simulink model "gm_Encoder_Zynq"  (R2018a)
settings: Solver=ode3  StartTime=0.0  StopTime=SimulationsDauer  RelTol=1e-3  EnableMultiTasking=on
undefined symbols (not defined in the file or in its folder): DiscIntNeverNeededParam, IncPerTurn, n_max, OverSamplingFactor, OverSamplingFactorInverse, Periode, Phase_Delay_A, Phase_Delay_B, PolePair, T_mech, TestDrehzahl_rpm
libraries: dspswit3 x2, powerlib_meascontrol x2, hdlmdlgenlib x1, simulink_extras x1, powerlib x1
(part 1 of 2)
settings Model: Creator=Wendel_ELSYS  LastModifiedBy=Wendel
settings DataIOCC: LimitDataPoints=on  SaveFormat=Array
settings OptimizationCC: BlockReduction=off  ConditionallyExecuteInputs=off  DefaultParameterBehavior=Inlined  LifeSpan=inf
settings DebuggingCC: AlgebraicLoopMsg=error  InheritedTsInSrcMsg=none  ParameterOverflowMsg=none  SFUnexpectedBacktrackingDiag=warning  SFNoUnconditionalDefaultTransitionDiag=warning  SFExecutionAtInitializationDiag=none
settings HardwareCC: ProdBitPerPointer=32  ProdBitPerSizeT=32  ProdBitPerPtrDiffT=32  ProdLargestAtomicFloat=None  ProdIntDivRoundTo=Undefined  ProdEndianess=Unspecified  ProdWordSize=32  ProdHWDeviceType=ASIC/FPGA->ASIC/FPGA  ProdEqTarget=off
settings ModelReferenceCC: PropagateSignalLabelsOutOfModel=off
settings CodeAppCC: StateflowObjectComments=on
settings GRTTargetCC: TargetLangStandard=C89/C90 (ANSI)  GeneratePreprocessorConditionals=Disable all
settings ConfigComp: CovMetricSettings=dw  CovHtmlReporting=on  CovSaveCumulativeToWorkspaceVar=on  CovSaveSingleToWorkspaceVar=on  CovExternalEMLEnable=off
settings SimscapeCC: SimscapeNormalizeSystem=off

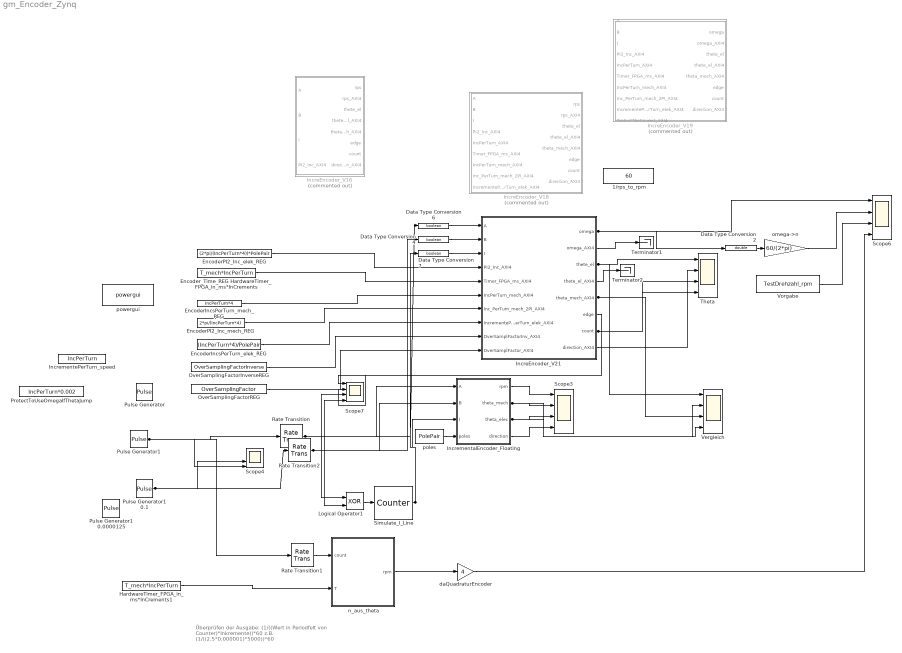
== system gm_Encoder_Zynq ==
  note: Überprüfen der Ausgabe:
      | (1/((Wert in Periodfelt von Counter)*Inkremente))*60
      | z.B. (1/((2.5*0.000001)*5000))*60
  1/rps_to_rpm : Constant  Value=60  OutDataTypeStr=double  SampleTime=T_mech
  Data Type Conversion2 : DataTypeConversion  OutDataTypeStr=double
  Data Type Conversion4 : DataTypeConversion  OutDataTypeStr=boolean
  Data Type Conversion6 : DataTypeConversion  OutDataTypeStr=boolean
  Data Type Conversion7 : DataTypeConversion  OutDataTypeStr=boolean
  "EncoderIncsPerTurn_elek_REG " : Constant  Value=(IncPerTurn*4)/PolePair  OutDataTypeStr=fixdt(0,16,0)  SampleTime=T_mech
  EncoderIncsPerTurn_mech_REG : Constant  Value=IncPerTurn*4  OutDataTypeStr=fixdt(0,16,0)  SampleTime=T_mech
  EncoderPI2_Inc_elek_REG : Constant  Value=(2*pi/(IncPerTurn*4))*PolePair  OutDataTypeStr=fixdt(0,24,24)  SampleTime=T_mech
  EncoderPI2_Inc_mech_REG : Constant  Value=2*pi/(IncPerTurn*4)  OutDataTypeStr=fixdt(0,24,24)  SampleTime=T_mech
  Encoder_Time_REG HardwareTimer_FPGA_in_ms*InCrements : Constant  Value=T_mech*IncPerTurn  OutDataTypeStr=fixdt(0,32,26)  SampleTime=T_mech
  HardwareTimer_FPGA_in_ms*InCrements1 : Constant  Value=T_mech*IncPerTurn  OutDataTypeStr=double  SampleTime=T_mech
  IncreEncoder_V16 : Subsystem  Commented=on  TreatAsAtomicUnit=on
  IncreEncoder_V18 : Subsystem  Commented=on  TreatAsAtomicUnit=on
  IncreEncoder_V19 : Subsystem  Commented=on  TreatAsAtomicUnit=on
  IncreEncoder_V21 : Subsystem  TreatAsAtomicUnit=on
  IncrementalEncoder_Floating : Subsystem
  IncrementePerTurn_speed : Constant  Value=IncPerTurn  OutDataTypeStr=fixdt(0,16,0)  SampleTime=T_mech
  Logical Operator1 : Logic  Operator=XOR  AllPortsSameDT=off  OutDataTypeStr=boolean
  OverSamplingFactorInverseREG : Constant  Value=OverSamplingFactorInverse  OutDataTypeStr=fixdt(0,16,15)  SampleTime=T_mech
  OverSamplingFactorREG : Constant  Value=OverSamplingFactor  OutDataTypeStr=fixdt(0,16,0)  SampleTime=T_mech
  ProtectToUseOmegaIfThetaJump : Constant  Value=IncPerTurn*0.002  OutDataTypeStr=uint16  SampleTime=T_mech
  Pulse Generator : DiscretePulseGenerator  PulseType=Time based  Period=0.01  PulseWidth=50  PhaseDelay=0.00000125  SampleTime=T_mech  VectorParams1D=off
  Pulse Generator1 : DiscretePulseGenerator  PulseType=Time based  Period=Periode  PulseWidth=50  PhaseDelay=Phase_Delay_A  SampleTime=T_mech  VectorParams1D=off
  Pulse Generator1 0.0000125 : DiscretePulseGenerator  PulseType=Time based  Period=0.01  PulseWidth=50  PhaseDelay=-0.00000125  SampleTime=T_mech  VectorParams1D=off
  Pulse Generator1 0.1 : DiscretePulseGenerator  PulseType=Time based  Period=Periode  PulseWidth=50  PhaseDelay=Phase_Delay_B  SampleTime=T_mech  VectorParams1D=off
  Rate Transition : RateTransition  Deterministic=off  OutPortSampleTime=T_mech
  Rate Transition1 : RateTransition  Deterministic=off  OutPortSampleTime=T_mech
  Rate Transition2 : RateTransition  Deterministic=off  OutPortSampleTime=T_mech
  Scope{3..4,6..7} (4 alike) : Scope  NumInputPorts=4
  Simulate_I_Line : dspswit3/Counter  Direction=Up  CountEvent=Either edge  CounterSize=User defined  MaxCount=IncPerTurn*4  InitialCount=0  Output=Hit  HitValue=IncPerTurn*4  ResetInput=off  SamplesPerFrame=1  Ts=1  CntDtype=double  HitDtype=Boolean
  Terminator1 : Terminator
  Terminator2 : Terminator
  Theta : Scope  NumInputPorts=4
  Vergleich : Scope  NumInputPorts=4
  Vorgabe : Constant  Value=TestDrehzahl_rpm
  "daQuadraturEncoder " : Gain  Gain=4
  n_aus_theta : Subsystem  TreatAsAtomicUnit=on
  omega->n : Gain  Gain=60/(2*pi)  OutDataTypeStr=double
  poles : Constant  Value=PolePair  OutDataTypeStr=uint8  SampleTime=-1
  powergui : powerlib/powergui  Priority=1  SimulationMode=Discrete  SampleTime=T_mech  frequency=60  Iterations=50  frequencyindice=0  Pbase=100e6  ErrMax=1e-4  UnitsV=kV  UnitsW=MW  buscounter=0  FunctionMessages=off  echomessages=off  EnableUseOfTLC=off  CurrentSourceSwitches=off  DisableSnubberDevices=off  DisableRonSwitches=off  DisableVfSwitches=off  DisplayEquations=off  SolverType=Tustin  Interpol=off  ExternalGateDelay=off  methode=off  Ts=0  x0status=blocks  SPID=off  SwTol=0  HookPort=off  RestoreLinks=warning  ResistiveCurrentMeasurement=off  Frange=[0:2:500]  Ylog=off  Xlog=on  ShowGrid=off  save=off  variable=ZData  structure=0  ZoomFFT=on  StartTime=0.0  cycles=1  DisplayStyle=1  fundamental=60  FreqAxis=off  MaxFrequency=1000  frequencyindicesteady=1  RmsSteady=1  display=off
  wires:
  OverSamplingFactorREG/1 -> IncreEncoder_V21/10(OverSamplFactor_AXI4)
  OverSamplingFactorInverseREG/1 -> IncreEncoder_V21/9(OverSamplFactorInv_AXI4)
  Vorgabe/1 -> Scope6/3
  "daQuadraturEncoder "/1 -> Scope6/4
  Pulse Generator1/1 -> Scope4/4, Rate Transition/1, Rate Transition1/1
  n_aus_theta/1(rpm) -> "daQuadraturEncoder "/1
  Rate Transition1/1 -> n_aus_theta/1(count)
  HardwareTimer_FPGA_in_ms*InCrements1/1 -> n_aus_theta/2(T)
  Data Type Conversion2/1 -> omega->n/1
  omega->n/1 -> Scope6/2
  "EncoderIncsPerTurn_elek_REG "/1 -> IncreEncoder_V21/8(IncrementePerTurn_elek_AXI4)
  EncoderPI2_Inc_mech_REG/1 -> IncreEncoder_V21/7(Inc_PerTurn_mech_2PI_AXI4)
  EncoderIncsPerTurn_mech_REG/1 -> IncreEncoder_V21/6(IncPerTurn_mech_AXI4)
  Encoder_Time_REG HardwareTimer_FPGA_in_ms*InCrements/1 -> IncreEncoder_V21/5(Timer_FPGA_ms_AXI4)
  IncreEncoder_V21/2(omega_AXI4) -> Terminator1/1
  IncreEncoder_V21/4(thete_el_AXI4) -> Terminator2/1
  IncreEncoder_V21/5(theta_mech_AXI4) -> Theta/3, Vergleich/3
  IncreEncoder_V21/3(thete_el) -> Vergleich/1, Theta/1
  EncoderPI2_Inc_elek_REG/1 -> IncreEncoder_V21/4(PI2_Inc_AXI4)
  poles/1 -> IncrementalEncoder_Floating/4(poles)
  IncrementalEncoder_Floating/4(direction) -> Scope3/4
  IncrementalEncoder_Floating/3(theta_elec) -> Scope3/3, Vergleich/2
  IncrementalEncoder_Floating/2(theta_mech) -> Scope3/2, Vergleich/4
  IncrementalEncoder_Floating/1(rpm) -> Scope3/1
  IncreEncoder_V21/7(count) -> Scope7/2, Theta/4
  IncreEncoder_V21/6(edge) -> Scope7/1
  IncreEncoder_V21/8(direction_AXI4) -> Theta/2
  IncreEncoder_V21/1(omega) -> Data Type Conversion2/1, Scope6/1
  Data Type Conversion7/1 -> IncreEncoder_V21/3(I)
  Data Type Conversion4/1 -> IncreEncoder_V21/2(B)
  Data Type Conversion6/1 -> IncreEncoder_V21/1(A)
  Rate Transition/1 -> Logical Operator1/1, IncrementalEncoder_Floating/1(A), Data Type Conversion6/1, Scope7/3
  Logical Operator1/1 -> Simulate_I_Line/1
  Simulate_I_Line/1 -> Data Type Conversion7/1, IncrementalEncoder_Floating/3(I)
  Rate Transition2/1 -> Data Type Conversion4/1, IncrementalEncoder_Floating/2(B), Scope7/4, Logical Operator1/2
  Pulse Generator1 0.1/1 -> Rate Transition2/1, Scope4/3

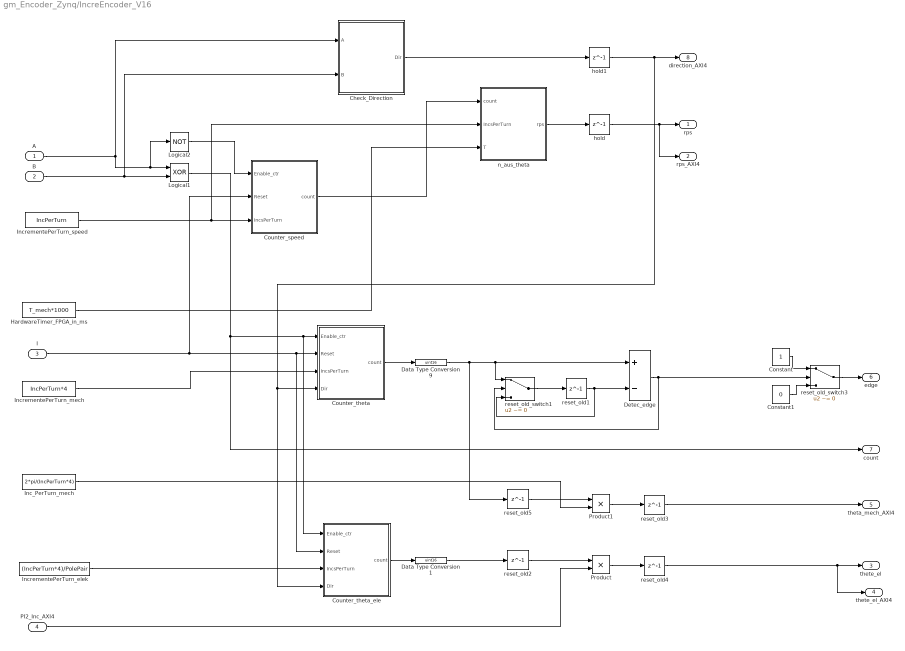
== system gm_Encoder_Zynq/IncreEncoder_V16 ==
  A : Inport
  B : Inport  Port=2
  I : Inport  Port=3
  PI2_Inc_AXI4 : Inport  Port=4
  Check_Direction : Subsystem  TreatAsAtomicUnit=on
  Constant : Constant  OutDataTypeStr=boolean  SampleTime=-1
  Constant1 : Constant  Value=0  OutDataTypeStr=boolean  SampleTime=-1
  Counter_speed : Subsystem  TreatAsAtomicUnit=on
  Counter_theta : Subsystem  TreatAsAtomicUnit=on
  Counter_theta_ele : Subsystem  TreatAsAtomicUnit=on
  Data Type Conversion1 : DataTypeConversion  OutDataTypeStr=uint16
  Data Type Conversion9 : DataTypeConversion  OutDataTypeStr=uint16
  Detec_edge : Sum  Inputs=+-  AccumDataTypeStr=uint8  OutDataTypeStr=uint8
  HardwareTimer_FPGA_in_ms : Constant  Value=T_mech*1000  OutDataTypeStr=fixdt(0,30,24)  SampleTime=T_mech
  Inc_PerTurn_mech : Constant  Value=2*pi/(IncPerTurn*4)  OutDataTypeStr=fixdt(0,24,24)  SampleTime=T_mech
  IncrementePerTurn_elek : Constant  Value=(IncPerTurn*4)/PolePair  OutDataTypeStr=fixdt(0,16,0)  SampleTime=T_mech
  IncrementePerTurn_mech : Constant  Value=IncPerTurn*4  OutDataTypeStr=fixdt(0,16,0)  SampleTime=T_mech
  IncrementePerTurn_speed : Constant  Value=IncPerTurn  OutDataTypeStr=fixdt(0,16,0)  SampleTime=T_mech
  Logical1 : Logic  Operator=XOR  AllPortsSameDT=off  OutDataTypeStr=boolean
  Logical2 : Logic  Operator=NOT  AllPortsSameDT=off  OutDataTypeStr=boolean
  Product : Product  OutDataTypeStr=fixdt(0,24,20)
  Product1 : Product  OutDataTypeStr=fixdt(0,24,20)
  hold : Delay  DelayLength=1
  hold1 : Delay  DelayLength=1
  n_aus_theta : Subsystem  TreatAsAtomicUnit=on
  reset_old{1..5} (5 alike) : Delay  DelayLength=1
  reset_old_switch1 : Switch  Criteria=u2 ~= 0
  reset_old_switch3 : Switch  Criteria=u2 ~= 0
  rps : Outport
  rps_AXI4 : Outport  Port=2
  thete_el : Outport  Port=3
  thete_el_AXI4 : Outport  Port=4
  theta_mech_AXI4 : Outport  Port=5
  edge : Outport  Port=6
  count : Outport  Port=7
  direction_AXI4 : Outport  Port=8
  wires:
  HardwareTimer_FPGA_in_ms/1 -> n_aus_theta/3(T)
  Logical2/1 -> Counter_speed/1(Enable_ctr)
  reset_old5/1 -> Product1/1
  reset_old2/1 -> Product/1
  Data Type Conversion1/1 -> reset_old2/1
  reset_old4/1 -> thete_el/1, thete_el_AXI4/1
  Counter_theta_ele/1(count) -> Data Type Conversion1/1
  PI2_Inc_AXI4/1 -> Product/2
  IncrementePerTurn_elek/1 -> Counter_theta_ele/3(IncsPerTurn)
  Data Type Conversion9/1 -> reset_old_switch1/1, Detec_edge/1, reset_old5/1
  n_aus_theta/1(rps) -> hold/1
  IncrementePerTurn_mech/1 -> Counter_theta/3(IncsPerTurn)
  Counter_speed/1(count) -> n_aus_theta/1(count)
  Logical1/1 -> Counter_theta/1(Enable_ctr), Counter_theta_ele/1(Enable_ctr), count/1
  Detec_edge/1 -> reset_old_switch1/2, reset_old_switch3/2
  Constant1/1 -> reset_old_switch3/3
  reset_old_switch3/1 -> edge/1
  Constant/1 -> reset_old_switch3/1
  Product/1 -> reset_old4/1
  Inc_PerTurn_mech/1 -> Product1/2
  Product1/1 -> reset_old3/1
  reset_old3/1 -> theta_mech_AXI4/1
  reset_old1/1 -> Detec_edge/2, reset_old_switch1/3
  reset_old_switch1/1 -> reset_old1/1
  Counter_theta/1(count) -> Data Type Conversion9/1
  hold1/1 -> direction_AXI4/1, Counter_theta/4(Dir), Counter_theta_ele/4(Dir)
  hold/1 -> rps/1, rps_AXI4/1
  Check_Direction/1(Dir) -> hold1/1
  IncrementePerTurn_speed/1 -> n_aus_theta/2(IncsPerTurn), Counter_speed/3(IncsPerTurn)
  I/1 -> Counter_theta/2(Reset), Counter_theta_ele/2(Reset), Counter_speed/2(Reset)
  B/1 -> Logical1/2, Check_Direction/2(B)
  A/1 -> Logical1/1, Logical2/1, Check_Direction/1(A)

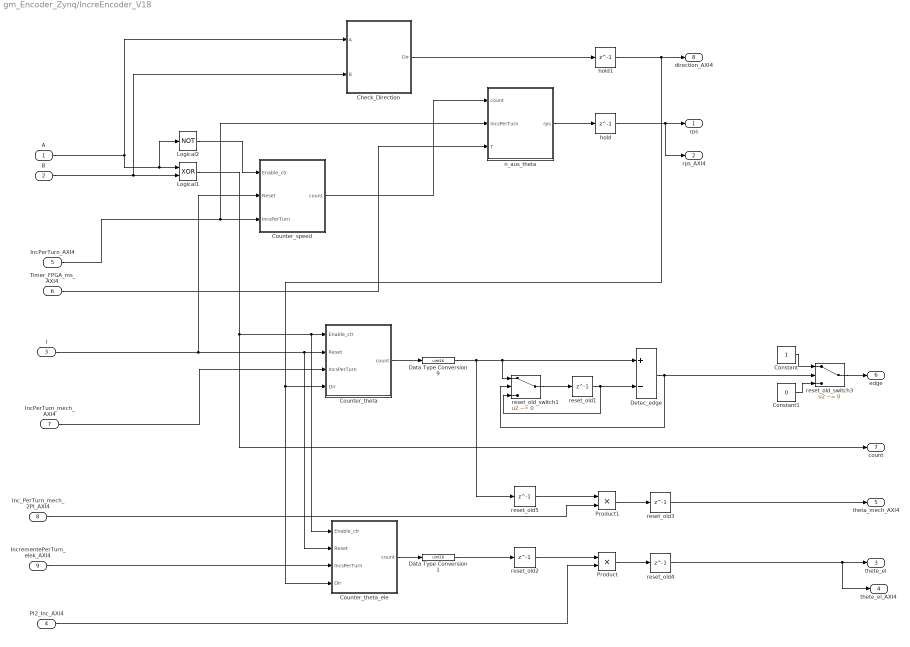
== system gm_Encoder_Zynq/IncreEncoder_V18 ==
  A : Inport
  B : Inport  Port=2
  I : Inport  Port=3
  PI2_Inc_AXI4 : Inport  Port=4
  IncPerTurn_AXI4 : Inport  Port=5
  Timer_FPGA_ms_AXI4 : Inport  Port=6
  IncPerTurn_mech_AXI4 : Inport  Port=7
  Inc_PerTurn_mech_2PI_AXI4 : Inport  Port=8
  IncrementePerTurn_elek_AXI4 : Inport  Port=9
  Check_Direction : Subsystem  TreatAsAtomicUnit=on
  Constant : Constant  OutDataTypeStr=boolean  SampleTime=-1
  Constant1 : Constant  Value=0  OutDataTypeStr=boolean  SampleTime=-1
  Counter_speed : Subsystem  TreatAsAtomicUnit=on
  Counter_theta : Subsystem  TreatAsAtomicUnit=on
  Counter_theta_ele : Subsystem  TreatAsAtomicUnit=on
  Data Type Conversion1 : DataTypeConversion  OutDataTypeStr=uint16
  Data Type Conversion9 : DataTypeConversion  OutDataTypeStr=uint16
  Detec_edge : Sum  Inputs=+-  AccumDataTypeStr=uint8  OutDataTypeStr=uint8
  Logical1 : Logic  Operator=XOR  AllPortsSameDT=off  OutDataTypeStr=boolean
  Logical2 : Logic  Operator=NOT  AllPortsSameDT=off  OutDataTypeStr=boolean
  Product : Product  OutDataTypeStr=fixdt(1,24,20)
  Product1 : Product  OutDataTypeStr=fixdt(1,24,20)
  hold : Delay  DelayLength=1
  hold1 : Delay  DelayLength=1
  n_aus_theta : Subsystem  TreatAsAtomicUnit=on
  reset_old{1..5} (5 alike) : Delay  DelayLength=1
  reset_old_switch1 : Switch  Criteria=u2 ~= 0
  reset_old_switch3 : Switch  Criteria=u2 ~= 0
  rps : Outport
  rps_AXI4 : Outport  Port=2
  thete_el : Outport  Port=3
  thete_el_AXI4 : Outport  Port=4
  theta_mech_AXI4 : Outport  Port=5
  edge : Outport  Port=6
  count : Outport  Port=7
  direction_AXI4 : Outport  Port=8
  wires:
  Timer_FPGA_ms_AXI4/1 -> n_aus_theta/3(T)
  Logical2/1 -> Counter_speed/1(Enable_ctr)
  reset_old5/1 -> Product1/1
  reset_old2/1 -> Product/1
  Data Type Conversion1/1 -> reset_old2/1
  reset_old4/1 -> thete_el/1, thete_el_AXI4/1
  Counter_theta_ele/1(count) -> Data Type Conversion1/1
  PI2_Inc_AXI4/1 -> Product/2
  IncrementePerTurn_elek_AXI4/1 -> Counter_theta_ele/3(IncsPerTurn)
  Data Type Conversion9/1 -> reset_old_switch1/1, Detec_edge/1, reset_old5/1
  n_aus_theta/1(rps) -> hold/1
  IncPerTurn_mech_AXI4/1 -> Counter_theta/3(IncsPerTurn)
  Counter_speed/1(count) -> n_aus_theta/1(count)
  Logical1/1 -> Counter_theta/1(Enable_ctr), Counter_theta_ele/1(Enable_ctr), count/1
  Detec_edge/1 -> reset_old_switch1/2, reset_old_switch3/2
  Constant1/1 -> reset_old_switch3/3
  reset_old_switch3/1 -> edge/1
  Constant/1 -> reset_old_switch3/1
  Product/1 -> reset_old4/1
  Inc_PerTurn_mech_2PI_AXI4/1 -> Product1/2
  Product1/1 -> reset_old3/1
  reset_old3/1 -> theta_mech_AXI4/1
  reset_old1/1 -> Detec_edge/2, reset_old_switch1/3
  reset_old_switch1/1 -> reset_old1/1
  Counter_theta/1(count) -> Data Type Conversion9/1
  hold1/1 -> direction_AXI4/1, Counter_theta/4(Dir), Counter_theta_ele/4(Dir)
  hold/1 -> rps/1, rps_AXI4/1
  Check_Direction/1(Dir) -> hold1/1
  IncPerTurn_AXI4/1 -> n_aus_theta/2(IncsPerTurn), Counter_speed/3(IncsPerTurn)
  I/1 -> Counter_theta/2(Reset), Counter_theta_ele/2(Reset), Counter_speed/2(Reset)
  B/1 -> Logical1/2, Check_Direction/2(B)
  A/1 -> Logical1/1, Logical2/1, Check_Direction/1(A)

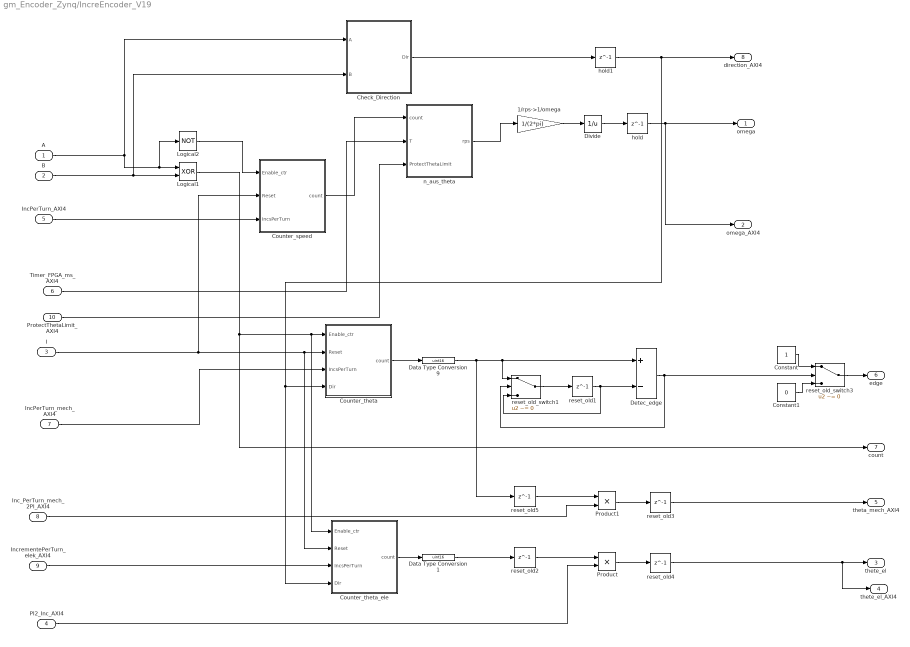
== system gm_Encoder_Zynq/IncreEncoder_V19 ==
  A : Inport
  B : Inport  Port=2
  I : Inport  Port=3
  PI2_Inc_AXI4 : Inport  Port=4
  IncPerTurn_AXI4 : Inport  Port=5
  Timer_FPGA_ms_AXI4 : Inport  Port=6
  IncPerTurn_mech_AXI4 : Inport  Port=7
  Inc_PerTurn_mech_2PI_AXI4 : Inport  Port=8
  IncrementePerTurn_elek_AXI4 : Inport  Port=9
  ProtectThetaLimit_AXI4 : Inport  Port=10
  1/rps->1/omega : Gain  Gain=1/(2*pi)  OutDataTypeStr=fixdt(1,24,18)
  Check_Direction : Subsystem  TreatAsAtomicUnit=on
  Constant : Constant  OutDataTypeStr=boolean  SampleTime=-1
  Constant1 : Constant  Value=0  OutDataTypeStr=boolean  SampleTime=-1
  Counter_speed : Subsystem  TreatAsAtomicUnit=on
  Counter_theta : Subsystem  TreatAsAtomicUnit=on
  Counter_theta_ele : Subsystem  TreatAsAtomicUnit=on
  Data Type Conversion1 : DataTypeConversion  OutDataTypeStr=uint16
  Data Type Conversion9 : DataTypeConversion  OutDataTypeStr=uint16
  Detec_edge : Sum  Inputs=+-  AccumDataTypeStr=uint8  OutDataTypeStr=uint8
  Divide : Math  Operator=reciprocal  OutDataTypeStr=fixdt(1,24,11)  RndMeth=Zero  SaturateOnIntegerOverflow=on
  Logical1 : Logic  Operator=XOR  AllPortsSameDT=off  OutDataTypeStr=boolean
  Logical2 : Logic  Operator=NOT  AllPortsSameDT=off  OutDataTypeStr=boolean
  Product : Product  OutDataTypeStr=fixdt(1,24,20)
  Product1 : Product  OutDataTypeStr=fixdt(1,24,20)
  hold : Delay  DelayLength=1
  hold1 : Delay  DelayLength=1
  n_aus_theta : Subsystem  TreatAsAtomicUnit=on
  reset_old{1..5} (5 alike) : Delay  DelayLength=1
  reset_old_switch1 : Switch  Criteria=u2 ~= 0
  reset_old_switch3 : Switch  Criteria=u2 ~= 0
  omega : Outport
  omega_AXI4 : Outport  Port=2
  thete_el : Outport  Port=3
  thete_el_AXI4 : Outport  Port=4
  theta_mech_AXI4 : Outport  Port=5
  edge : Outport  Port=6
  count : Outport  Port=7
  direction_AXI4 : Outport  Port=8
  wires:
  ProtectThetaLimit_AXI4/1 -> n_aus_theta/3(ProtectThetaLimit)
  1/rps->1/omega/1 -> Divide/1
  Divide/1 -> hold/1
  Timer_FPGA_ms_AXI4/1 -> n_aus_theta/2(T)
  Logical2/1 -> Counter_speed/1(Enable_ctr)
  reset_old5/1 -> Product1/1
  reset_old2/1 -> Product/1
  Data Type Conversion1/1 -> reset_old2/1
  reset_old4/1 -> thete_el/1, thete_el_AXI4/1
  Counter_theta_ele/1(count) -> Data Type Conversion1/1
  PI2_Inc_AXI4/1 -> Product/2
  IncrementePerTurn_elek_AXI4/1 -> Counter_theta_ele/3(IncsPerTurn)
  Data Type Conversion9/1 -> reset_old_switch1/1, Detec_edge/1, reset_old5/1
  n_aus_theta/1(rps) -> 1/rps->1/omega/1
  IncPerTurn_mech_AXI4/1 -> Counter_theta/3(IncsPerTurn)
  Counter_speed/1(count) -> n_aus_theta/1(count)
  Logical1/1 -> Counter_theta/1(Enable_ctr), Counter_theta_ele/1(Enable_ctr), count/1
  Detec_edge/1 -> reset_old_switch1/2, reset_old_switch3/2
  Constant1/1 -> reset_old_switch3/3
  reset_old_switch3/1 -> edge/1
  Constant/1 -> reset_old_switch3/1
  Product/1 -> reset_old4/1
  Inc_PerTurn_mech_2PI_AXI4/1 -> Product1/2
  Product1/1 -> reset_old3/1
  reset_old3/1 -> theta_mech_AXI4/1
  reset_old1/1 -> Detec_edge/2, reset_old_switch1/3
  reset_old_switch1/1 -> reset_old1/1
  Counter_theta/1(count) -> Data Type Conversion9/1
  hold1/1 -> direction_AXI4/1, Counter_theta/4(Dir), Counter_theta_ele/4(Dir)
  hold/1 -> omega/1, omega_AXI4/1
  Check_Direction/1(Dir) -> hold1/1
  IncPerTurn_AXI4/1 -> Counter_speed/3(IncsPerTurn)
  I/1 -> Counter_theta/2(Reset), Counter_theta_ele/2(Reset), Counter_speed/2(Reset)
  B/1 -> Logical1/2, Check_Direction/2(B)
  A/1 -> Logical1/1, Logical2/1, Check_Direction/1(A)

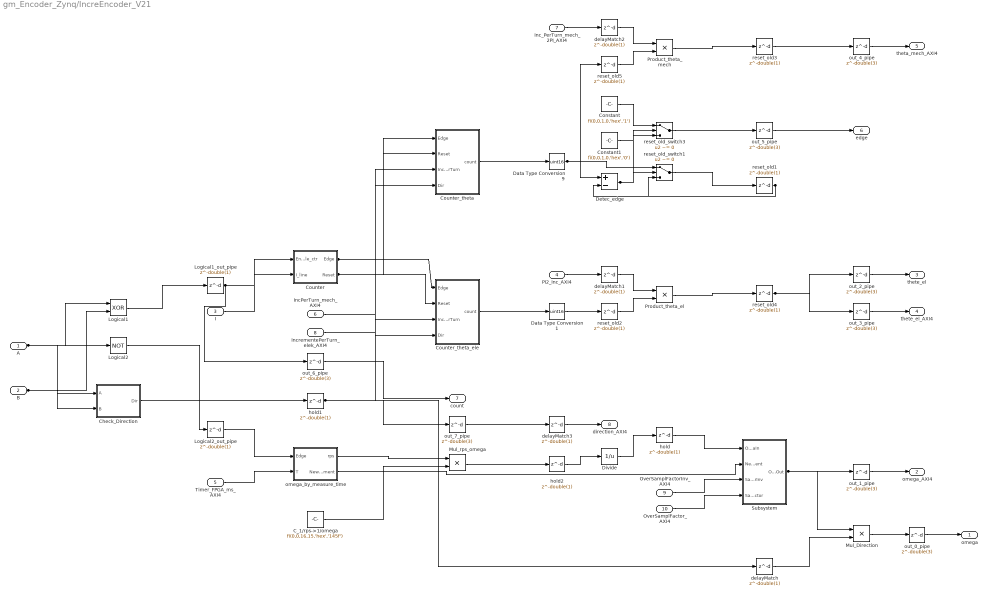
== system gm_Encoder_Zynq/IncreEncoder_V21 ==
  A : Inport  OutDataTypeStr=boolean  PortDimensions=1  SampleTime=2e-08
  B : Inport  Port=2  OutDataTypeStr=boolean  PortDimensions=1  SampleTime=2e-08
  I : Inport  Port=3  OutDataTypeStr=boolean  PortDimensions=1  SampleTime=2e-08
  PI2_Inc_AXI4 : Inport  Port=4  OutDataTypeStr=fixdt(0, 24, 24)  PortDimensions=1  SampleTime=2e-08
  Timer_FPGA_ms_AXI4 : Inport  Port=5  OutDataTypeStr=fixdt(0, 32, 26)  PortDimensions=1  SampleTime=2e-08
  IncPerTurn_mech_AXI4 : Inport  Port=6  OutDataTypeStr=uint16  PortDimensions=1  SampleTime=2e-08
  Inc_PerTurn_mech_2PI_AXI4 : Inport  Port=7  OutDataTypeStr=fixdt(0, 24, 24)  PortDimensions=1  SampleTime=2e-08
  IncrementePerTurn_elek_AXI4 : Inport  Port=8  OutDataTypeStr=uint16  PortDimensions=1  SampleTime=2e-08
  OverSamplFactorInv_AXI4 : Inport  Port=9  OutDataTypeStr=fixdt(0, 16, 15)  PortDimensions=1  SampleTime=2e-08
  OverSamplFactor_AXI4 : Inport  Port=10  OutDataTypeStr=uint16  PortDimensions=1  SampleTime=2e-08
  C_1/rps->1/omega : Constant  Value=fi(0,0,16,15,'hex','145f')  OutDataTypeStr=fixdt(0, 16, 15)  SampleTime=-1
  Check_Direction : Subsystem
  Constant : Constant  Value=fi(0,0,1,0,'hex','1')  OutDataTypeStr=boolean  SampleTime=-1
  Constant1 : Constant  Value=fi(0,0,1,0,'hex','0')  OutDataTypeStr=boolean  SampleTime=-1
  Counter : Subsystem
  Counter_theta : Subsystem
  Counter_theta_ele : Subsystem
  Data Type Conversion1 : DataTypeConversion  OutDataTypeStr=uint16  SampleTime=2e-08
  Data Type Conversion9 : DataTypeConversion  OutDataTypeStr=uint16  SampleTime=2e-08
  Detec_edge : Sum  Inputs=+-  AccumDataTypeStr=uint8  OutDataTypeStr=uint8  SampleTime=2e-08
  Divide : Math  Operator=reciprocal  OutDataTypeStr=fixdt(1,24,11)  RndMeth=Zero  SaturateOnIntegerOverflow=on
  Logical1 : Logic  Operator=XOR  AllPortsSameDT=off  OutDataTypeStr=boolean  SampleTime=2e-08
  Logical1_out_pipe : Delay  DelayLength=double(1)  InitialCondition=0  InputProcessing=Inherited  SampleTime=2e-08
  Logical2 : Logic  Operator=NOT  Inputs=1  AllPortsSameDT=off  OutDataTypeStr=boolean  SampleTime=2e-08
  Logical2_out_pipe : Delay  DelayLength=double(1)  InitialCondition=0  InputProcessing=Inherited  SampleTime=2e-08
  Mul_Direction : Product  Inputs=**  OutDataTypeStr=fixdt(1, 24, 11)  SampleTime=2e-08  SaturateOnIntegerOverflow=on  RndMeth=Zero
  Mul_rps_omega : Product  Inputs=**  OutDataTypeStr=fixdt(0, 32, 26)  SampleTime=2e-08  SaturateOnIntegerOverflow=on  RndMeth=Zero
  Product_theta_el : Product  Inputs=**  OutDataTypeStr=fixdt(1, 24, 20)  SampleTime=2e-08
  Product_theta_mech : Product  Inputs=**  OutDataTypeStr=fixdt(1, 24, 20)  SampleTime=2e-08
  Subsystem : Subsystem
  delayMatch{,1..3} (4 alike) : Delay  DelayLength=double(1)  InitialCondition=0  InputProcessing=Inherited  SampleTime=2e-08
  hold : Delay  DelayLength=double(1)  InitialCondition=0  InputProcessing=Inherited  SampleTime=2e-08
  hold1 : Delay  DelayLength=double(1)  InitialCondition=0  InputProcessing=Inherited  SampleTime=2e-08
  hold2 : Delay  DelayLength=double(1)  InitialCondition=0  InputProcessing=Inherited  SampleTime=2e-08
  omega_by_measure_time : Subsystem
  out_0_pipe : Delay  DelayLength=double(3)  InitialCondition=0  InputProcessing=Inherited  SampleTime=2e-08
  out_1_pipe : Delay  DelayLength=double(3)  InitialCondition=0  InputProcessing=Inherited  SampleTime=2e-08
  out_2_pipe : Delay  DelayLength=double(3)  InitialCondition=0  InputProcessing=Inherited  SampleTime=2e-08
  out_3_pipe : Delay  DelayLength=double(3)  InitialCondition=0  InputProcessing=Inherited  SampleTime=2e-08
  out_4_pipe : Delay  DelayLength=double(3)  InitialCondition=0  InputProcessing=Inherited  SampleTime=2e-08
  out_5_pipe : Delay  DelayLength=double(3)  InitialCondition=0  InputProcessing=Inherited  SampleTime=2e-08
  out_6_pipe : Delay  DelayLength=double(3)  InitialCondition=0  InputProcessing=Inherited  SampleTime=2e-08
  out_7_pipe : Delay  DelayLength=double(3)  InitialCondition=0  InputProcessing=Inherited  SampleTime=2e-08
  reset_old{1..5} (5 alike) : Delay  DelayLength=double(1)  InitialCondition=0  InputProcessing=Inherited  SampleTime=2e-08
  reset_old_switch1 : Switch  Criteria=u2 ~= 0  Threshold=double(0)  OutDataTypeStr=uint16  SampleTime=2e-08
  reset_old_switch3 : Switch  Criteria=u2 ~= 0  Threshold=double(0)  OutDataTypeStr=boolean  SampleTime=2e-08
  omega : Outport
  omega_AXI4 : Outport  Port=2
  thete_el : Outport  Port=3
  thete_el_AXI4 : Outport  Port=4
  theta_mech_AXI4 : Outport  Port=5
  edge : Outport  Port=6
  count : Outport  Port=7
  direction_AXI4 : Outport  Port=8
  wires:
  A/1 -> Logical2/1, Logical1/1, Check_Direction/1(A)
  B/1 -> Logical1/2, Check_Direction/2(B)
  I/1 -> Counter/2(I_line)
  delayMatch1/1 -> Product_theta_el/1
  Timer_FPGA_ms_AXI4/1 -> omega_by_measure_time/2(T)
  IncPerTurn_mech_AXI4/1 -> Counter_theta/3(IncsPerTurn)
  delayMatch2/1 -> Product_theta_mech/1
  IncrementePerTurn_elek_AXI4/1 -> Counter_theta_ele/3(IncsPerTurn)
  OverSamplFactorInv_AXI4/1 -> Subsystem/3(SamplingFactorInv)
  OverSamplFactor_AXI4/1 -> Subsystem/4(SamplingFactor)
  C_1/rps->1/omega/1 -> Mul_rps_omega/2
  Check_Direction/1(Dir) -> hold1/1
  Constant/1 -> reset_old_switch3/1
  Constant1/1 -> reset_old_switch3/3
  Counter/1(Edge) -> Counter_theta_ele/1(Edge), Counter_theta/1(Edge)
  Counter/2(Reset) -> Counter_theta_ele/2(Reset), Counter_theta/2(Reset)
  Counter_theta/1(count) -> Data Type Conversion9/1
  Counter_theta_ele/1(count) -> Data Type Conversion1/1
  Data Type Conversion1/1 -> reset_old2/1
  Data Type Conversion9/1 -> reset_old5/1, reset_old_switch1/1, Detec_edge/1
  Divide/1 -> hold/1
  Logical1_out_pipe/1 -> out_6_pipe/1, Counter/1(Enable_ctr)
  Logical2_out_pipe/1 -> omega_by_measure_time/1(Edge)
  Mul_Direction/1 -> out_0_pipe/1
  Mul_rps_omega/1 -> hold2/1
  Product_theta_el/1 -> reset_old4/1
  Product_theta_mech/1 -> reset_old3/1
  Subsystem/1(OmegaOut) -> Mul_Direction/1, out_1_pipe/1
  hold/1 -> Subsystem/1("OmegaIn ")
  delayMatch/1 -> Mul_Direction/2
  hold2/1 -> Divide/1
  omega_by_measure_time/1(rps) -> Mul_rps_omega/1
  omega_by_measure_time/2(NewMeasurement) -> Subsystem/2(NewMeasurement)
  reset_old2/1 -> Product_theta_el/2
  reset_old3/1 -> out_4_pipe/1
  reset_old4/1 -> out_3_pipe/1, out_2_pipe/1
  reset_old5/1 -> Product_theta_mech/2
  reset_old_switch3/1 -> out_5_pipe/1
  out_0_pipe/1 -> omega/1
  out_1_pipe/1 -> omega_AXI4/1
  out_2_pipe/1 -> thete_el/1
  out_3_pipe/1 -> thete_el_AXI4/1
  out_4_pipe/1 -> theta_mech_AXI4/1
  out_5_pipe/1 -> edge/1
  out_6_pipe/1 -> count/1
  delayMatch3/1 -> direction_AXI4/1
  Logical1/1 -> Logical1_out_pipe/1
  Logical2/1 -> Logical2_out_pipe/1
  hold1/1 -> delayMatch/1, out_7_pipe/1, Counter_theta_ele/4(Dir), Counter_theta/4(Dir)
  PI2_Inc_AXI4/1 -> delayMatch1/1
  Inc_PerTurn_mech_2PI_AXI4/1 -> delayMatch2/1
  out_7_pipe/1 -> delayMatch3/1
  reset_old_switch1/1 -> reset_old1/1
  reset_old1/1 -> reset_old_switch1/3, Detec_edge/2
  Detec_edge/1 -> reset_old_switch1/2, reset_old_switch3/2

== system gm_Encoder_Zynq/IncrementalEncoder_Floating ==
  A : Inport
  B : Inport  Port=2
  I : Inport  Port=3
  poles : Inport  Port=4
  Add : Sum  Inputs=+-  OutDataTypeStr=fixdt(1,16,0)
  Counter3 : dspswit3/Counter  Direction=Up  CountEvent=Either edge  CounterSize=User defined  MaxCount=IncPerTurn*4  InitialCount=0  Output=Count  HitValue=32  ResetInput=on  SamplesPerFrame=1  Ts=1  CntDtype=double  HitDtype=Logical
  CutTheta_0_2PI : Subsystem
  Edge Detector2 : powerlib_meascontrol/Logic/Edge Detector  model=Rising  ic=0  Ts=-1
      settings: SourceProductName=Simscape Power Systems  SourceProductBaseCode=PS
  Edge Detector3 : powerlib_meascontrol/Logic/Edge Detector  model=Rising  ic=0  Ts=-1
      settings: SourceProductName=Simscape Power Systems  SourceProductBaseCode=PS
  Logical Operator1 : Logic  Operator=XOR  AllPortsSameDT=off  OutDataTypeStr=boolean
  Logical Operator3 : Logic  AllPortsSameDT=off  OutDataTypeStr=boolean
  Logical Operator4 : Logic  Operator=NOT  AllPortsSameDT=off  OutDataTypeStr=boolean
  Logical Operator5 : Logic  AllPortsSameDT=off  OutDataTypeStr=boolean
  Logical Operator6 : Logic  Operator=NOT  AllPortsSameDT=off  OutDataTypeStr=boolean
  Product : Product
  S-R Flip-Flop1 : simulink_extras/Flip Flops/S-R Flip-Flop  initial_condition=0
  Scope1 : Scope  NumInputPorts=4
  cut_theta_2pi : Gain  Gain=(2*pi)/IncPerTurn
  cut_theta_2pi1 : Gain  Gain=(2*pi)/IncPerTurn
  n_aus_theta_v4 : Subsystem
  rpm : Outport
  theta_mech : Outport  Port=2
  theta_elec : Outport  Port=3
  direction : Outport  Port=4
  wires:
  Add/1 -> direction/1
  B/1 -> Logical Operator1/2, Logical Operator4/1, Edge Detector3/1
  A/1 -> Logical Operator1/1, Edge Detector2/1, Logical Operator6/1
  S-R Flip-Flop1/2 -> Add/2
  S-R Flip-Flop1/1 -> Add/1
  Logical Operator5/1 -> S-R Flip-Flop1/2
  Logical Operator6/1 -> Logical Operator5/2
  Edge Detector3/1 -> Logical Operator5/1
  Logical Operator3/1 -> S-R Flip-Flop1/1
  Logical Operator4/1 -> Logical Operator3/2
  Edge Detector2/1 -> Logical Operator3/1
  CutTheta_0_2PI/1(Out1) -> theta_elec/1
  cut_theta_2pi1/1 -> CutTheta_0_2PI/1(In1)
  poles/1 -> Product/2
  Product/1 -> cut_theta_2pi1/1
  cut_theta_2pi/1 -> theta_mech/1, n_aus_theta_v4/1(theta), Scope1/2
  Logical Operator1/1 -> Counter3/1, Scope1/4
  n_aus_theta_v4/1(n) -> rpm/1
  Counter3/1 -> Scope1/1, Product/1, cut_theta_2pi/1
  I/1 -> Counter3/2

== system gm_Encoder_Zynq/n_aus_theta ==
  count : Inport
  T : Inport  Port=2
  1/rps->1/omega : Gain  Gain=1/(2*pi)  OutDataTypeStr=double
  Add : Sum  Inputs=+-
  Add1 : Sum
  Constant : Constant  Value=0  OutDataTypeStr=double  SampleTime=-1
  Constant1 : Constant  Value=0  OutDataTypeStr=double  SampleTime=-1
  Constant2 : Constant  Value=0  OutDataTypeStr=double  SampleTime=-1
  Divide1 : Product  Inputs=/
  ProtectOverflow_T_count : Switch  Threshold=50
  ProtectOverflow_rps : Switch  Threshold=50  OutDataTypeStr=double
  Scope1 : Scope  NumInputPorts=4
  Scope2 : Scope  NumInputPorts=4
  T_count : Delay  DelayLength=1
  T_count_switch : Switch  Criteria=u2 ~= 0
  count_old : Delay  DelayLength=1
  count_old_switch : Switch  Criteria=u2 ~= 0
  speed_old : Delay  DelayLength=1
  speed_old_switch : Switch  Criteria=u2 ~= 0
  rpm : Outport
  wires:
  Divide1/1 -> rpm/1
  1/rps->1/omega/1 -> Divide1/1
  T_count_switch/1 -> ProtectOverflow_T_count/3, ProtectOverflow_T_count/2, Scope1/2, ProtectOverflow_rps/2
  count/1 -> count_old_switch/1, Add/1
  Add1/1 -> T_count_switch/3, speed_old_switch/1, Scope2/2
  T_count/1 -> Add1/2, Scope1/4
  ProtectOverflow_T_count/1 -> T_count/1
  T/1 -> Add1/1, Scope2/4
  speed_old/1 -> speed_old_switch/3
  speed_old_switch/1 -> speed_old/1, Scope2/3, ProtectOverflow_rps/3
  Constant2/1 -> ProtectOverflow_rps/1
  ProtectOverflow_rps/1 -> Scope2/1, 1/rps->1/omega/1
  Constant1/1 -> ProtectOverflow_T_count/1
  Add/1 -> T_count_switch/2, Scope1/1, count_old_switch/2, speed_old_switch/2
  Constant/1 -> T_count_switch/1
  count_old/1 -> Add/2, count_old_switch/3
  count_old_switch/1 -> count_old/1

== system gm_Encoder_Zynq/IncreEncoder_V16/Check_Direction ==
  A : Inport
  B : Inport  Port=2
  Add : Sum  Inputs=+-  AccumDataTypeStr=fixdt(1,4,0)  OutDataTypeStr=fixdt(1,4,0)
  Add1 : Sum  Inputs=+-  AccumDataTypeStr=fixdt(1,4,0)  OutDataTypeStr=fixdt(1,4,0)
  Add2 : Sum  AccumDataTypeStr=fixdt(1,4,0)  OutDataTypeStr=fixdt(1,4,0)
  Change : Sum  AccumDataTypeStr=fixdt(1,4,0)  OutDataTypeStr=fixdt(1,4,0)
  Change1 : Delay  DelayLength=1
  Save_Direction : Switch  Criteria=u2 ~= 0  Threshold=0.1  OutDataTypeStr=Inherit: Inherit via back propagation
  Scope6 : Scope  NumInputPorts=4
  T_count_switch : Switch  Threshold=1  OutDataTypeStr=Inherit: Inherit via back propagation
  TrnLeft : Sum  Inputs=+-  AccumDataTypeStr=fixdt(1,4,0)  OutDataTypeStr=fixdt(1,4,0)
  TrnRight : Sum  Inputs=+-  AccumDataTypeStr=fixdt(1,4,0)  OutDataTypeStr=fixdt(1,4,0)
  TurnLeft : Constant  Value=-1  OutDataTypeStr=fixdt(1,4,0)  SampleTime=-1
  TurnRight : Constant  OutDataTypeStr=fixdt(1,4,0)  SampleTime=-1
  count_old : Delay  DelayLength=1
  count_old1 : Delay  DelayLength=1
  count_old2 : Delay  DelayLength=1
  count_old_switch : Switch  Criteria=u2 ~= 0  OutDataTypeStr=Inherit: Inherit via back propagation
  count_old_switch1 : Switch  Criteria=u2 ~= 0  OutDataTypeStr=Inherit: Inherit via back propagation
  new_value : Delay  DelayLength=1
  nothing : Constant  Value=0  OutDataTypeStr=fixdt(1,4,0)  SampleTime=-1
  nothing1 : Constant  Value=0  OutDataTypeStr=fixdt(1,4,0)  SampleTime=-1
  speed_old_switch : Switch  Threshold=1  OutDataTypeStr=Inherit: Inherit via back propagation
  Dir : Outport
  wires:
  count_old2/1 -> Dir/1, Save_Direction/3
  Change1/1 -> Save_Direction/2, Scope6/3
  Change/1 -> Change1/1
  Add2/1 -> new_value/1, Scope6/4
  speed_old_switch/1 -> Add2/2, Change/2
  nothing1/1 -> T_count_switch/3
  nothing/1 -> speed_old_switch/3
  TurnLeft/1 -> speed_old_switch/1
  TrnLeft/1 -> Scope6/2, speed_old_switch/2
  new_value/1 -> Save_Direction/1
  TrnRight/1 -> T_count_switch/2, Scope6/1
  Add1/1 -> count_old_switch1/2, TrnLeft/1
  count_old1/1 -> Add1/2, count_old_switch1/3
  count_old_switch1/1 -> count_old1/1
  B/1 -> count_old_switch1/1, Add1/1, TrnRight/2
  Save_Direction/1 -> count_old2/1
  T_count_switch/1 -> Add2/1, Change/1
  Add/1 -> count_old_switch/2, TrnRight/1
  TurnRight/1 -> T_count_switch/1
  count_old/1 -> Add/2, count_old_switch/3
  count_old_switch/1 -> count_old/1
  A/1 -> count_old_switch/1, Add/1, TrnLeft/2

== system gm_Encoder_Zynq/IncreEncoder_V16/Counter_speed ==
  note: Count
  note: Reset
  note: Check if count is to big
  note: Check if count is to small
  note: 1 for one cycle if edge recognized
  Enable_ctr : Inport
  Reset : Inport  Port=2
  IncsPerTurn : Inport  Port=3
  Add1 : Sum  AccumDataTypeStr=int16  OutDataTypeStr=uint16
  Constant1 : Constant  Value=0  OutDataTypeStr=uint16  SampleTime=-1
  Constant2 : Constant  OutDataTypeStr=int8  SampleTime=-1
  Constant3 : Constant  Value=0  OutDataTypeStr=int8  SampleTime=-1
  Constant4 : Constant  Value=10  OutDataTypeStr=uint16  SampleTime=-1
  Detec_edge : Sum  Inputs=+-  AccumDataTypeStr=int8  OutDataTypeStr=int8
  Relational Operator : RelationalOperator  OutDataTypeStr=boolean  RndMeth=Nearest
  Reset_flag : Sum  Inputs=+-  AccumDataTypeStr=uint8  OutDataTypeStr=uint8
  Reset_when_overflow : Sum
  Resett_switch1 : Switch  Criteria=u2 ~= 0
  Resett_switch2 : Switch  Criteria=u2 ~= 0
  reset_old{,1..3} (4 alike) : Delay  DelayLength=1
  reset_old_switch : Switch  Criteria=u2 ~= 0
  reset_old_switch1 : Switch  Criteria=u2 ~= 0
  speed_old_switch1 : Switch  Threshold=1
  count : Outport
  wires:
  reset_old3/1 -> Relational Operator/2
  Resett_switch2/1 -> Resett_switch1/3
  IncsPerTurn/1 -> Reset_when_overflow/2
  Constant1/1 -> Resett_switch1/1, Resett_switch2/1
  Relational Operator/1 -> Resett_switch1/2
  Resett_switch1/1 -> reset_old2/1
  Reset_when_overflow/1 -> reset_old3/1
  Constant4/1 -> Reset_when_overflow/1
  Constant2/1 -> speed_old_switch1/1
  Constant3/1 -> speed_old_switch1/3
  speed_old_switch1/1 -> Add1/1
  reset_old2/1 -> count/1, Add1/2, Relational Operator/1
  Add1/1 -> Resett_switch2/3
  Detec_edge/1 -> reset_old_switch1/2, speed_old_switch1/2  "1 for one cycle if edge recognized"
  reset_old1/1 -> Detec_edge/2, reset_old_switch1/3
  reset_old_switch1/1 -> reset_old1/1
  Enable_ctr/1 -> reset_old_switch1/1, Detec_edge/1
  Reset_flag/1 -> Resett_switch2/2, reset_old_switch/2
  reset_old/1 -> Reset_flag/2, reset_old_switch/3
  reset_old_switch/1 -> reset_old/1
  Reset/1 -> reset_old_switch/1, Reset_flag/1

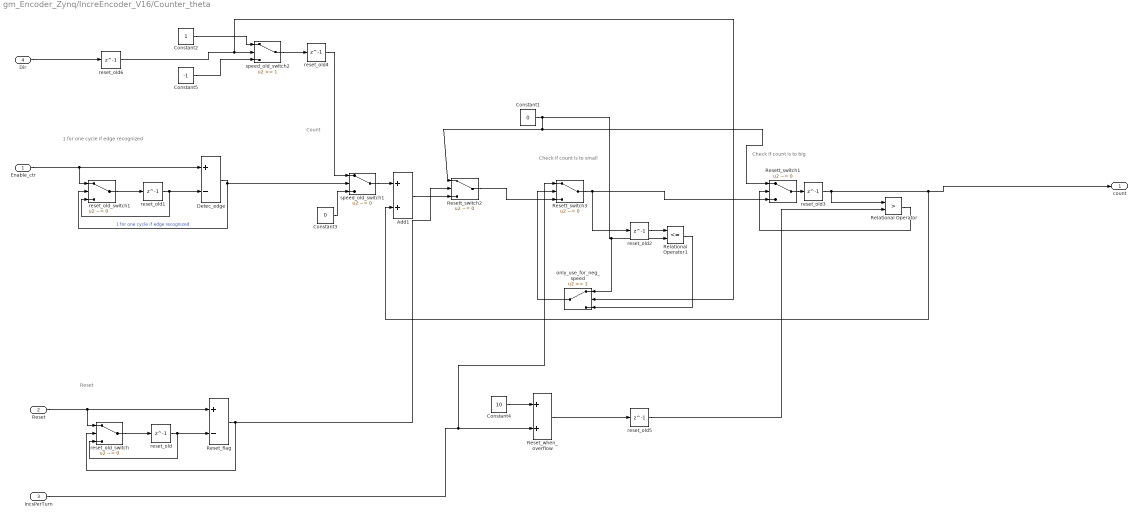
== system gm_Encoder_Zynq/IncreEncoder_V16/Counter_theta ==
  note: Check if count is to small
  note: Check if count is to big
  note: Count
  note: Reset
  note: 1 for one cycle if edge recognized
  Enable_ctr : Inport
  Reset : Inport  Port=2
  IncsPerTurn : Inport  Port=3
  Dir : Inport  Port=4
  Add1 : Sum  AccumDataTypeStr=int16  OutDataTypeStr=int16
  Constant1 : Constant  Value=0  OutDataTypeStr=int16  SampleTime=-1
  Constant2 : Constant  OutDataTypeStr=int16  SampleTime=-1
  Constant3 : Constant  Value=0  OutDataTypeStr=int16  SampleTime=-1
  Constant4 : Constant  Value=10  OutDataTypeStr=int16  SampleTime=-1
  Constant5 : Constant  Value=-1  OutDataTypeStr=int16  SampleTime=-1
  Detec_edge : Sum  Inputs=+-  AccumDataTypeStr=int8  OutDataTypeStr=int8
  Relational Operator : RelationalOperator  Operator=>  OutDataTypeStr=boolean  RndMeth=Nearest
  Relational Operator1 : RelationalOperator  Operator=<=  OutDataTypeStr=boolean  RndMeth=Nearest
  Reset_flag : Sum  Inputs=+-  AccumDataTypeStr=uint8  OutDataTypeStr=uint8
  Reset_when_overflow : Sum  OutDataTypeStr=int16
  Resett_switch1 : Switch  Criteria=u2 ~= 0  OutDataTypeStr=int16
  Resett_switch2 : Switch  Criteria=u2 ~= 0  OutDataTypeStr=int16
  Resett_switch3 : Switch  Criteria=u2 ~= 0  OutDataTypeStr=int16
  only_use_for_neg_speed : Switch  Threshold=1
  reset_old{,1..6} (7 alike) : Delay  DelayLength=1
  reset_old_switch : Switch  Criteria=u2 ~= 0
  reset_old_switch1 : Switch  Criteria=u2 ~= 0
  speed_old_switch1 : Switch  Criteria=u2 ~= 0
  speed_old_switch2 : Switch  Threshold=1
  count : Outport
  wires:
  reset_old6/1 -> speed_old_switch2/2, only_use_for_neg_speed/2
  reset_old5/1 -> Relational Operator/2
  reset_old4/1 -> speed_old_switch1/1
  only_use_for_neg_speed/1 -> Resett_switch3/2
  Relational Operator1/1 -> only_use_for_neg_speed/3
  reset_old2/1 -> Relational Operator1/1
  Resett_switch2/1 -> Resett_switch3/3
  Resett_switch3/1 -> Resett_switch1/3, reset_old2/1
  Constant1/1 -> Relational Operator1/2, only_use_for_neg_speed/1, Resett_switch1/1, Resett_switch2/1
  Relational Operator/1 -> Resett_switch1/2
  Resett_switch1/1 -> reset_old3/1
  reset_old3/1 -> Relational Operator/1, count/1, Add1/2
  speed_old_switch2/1 -> reset_old4/1
  Constant5/1 -> speed_old_switch2/3
  Dir/1 -> reset_old6/1
  IncsPerTurn/1 -> Reset_when_overflow/2, Resett_switch3/1
  Reset_when_overflow/1 -> reset_old5/1
  Constant4/1 -> Reset_when_overflow/1
  Constant2/1 -> speed_old_switch2/1
  Constant3/1 -> speed_old_switch1/3
  speed_old_switch1/1 -> Add1/1
  Add1/1 -> Resett_switch2/3
  Detec_edge/1 -> reset_old_switch1/2, speed_old_switch1/2  "1 for one cycle if edge recognized"
  reset_old1/1 -> Detec_edge/2, reset_old_switch1/3
  reset_old_switch1/1 -> reset_old1/1
  Enable_ctr/1 -> reset_old_switch1/1, Detec_edge/1
  Reset_flag/1 -> Resett_switch2/2, reset_old_switch/2
  reset_old/1 -> Reset_flag/2, reset_old_switch/3
  reset_old_switch/1 -> reset_old/1
  Reset/1 -> reset_old_switch/1, Reset_flag/1

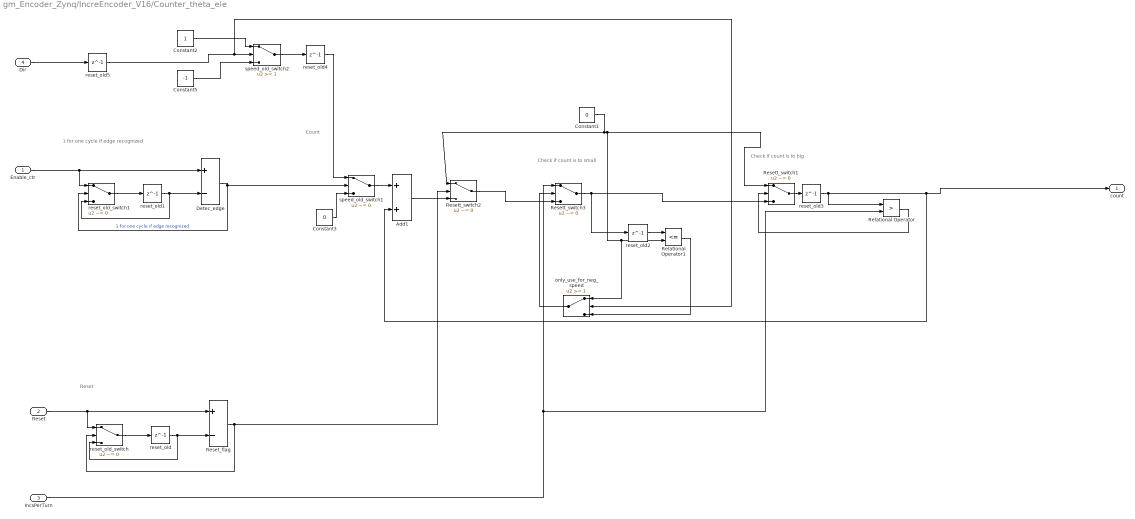
== system gm_Encoder_Zynq/IncreEncoder_V16/Counter_theta_ele ==
  note: Check if count is to small
  note: Check if count is to big
  note: Count
  note: Reset
  note: 1 for one cycle if edge recognized
  Enable_ctr : Inport
  Reset : Inport  Port=2
  IncsPerTurn : Inport  Port=3
  Dir : Inport  Port=4
  Add1 : Sum  AccumDataTypeStr=int16  OutDataTypeStr=int16
  Constant1 : Constant  Value=0  OutDataTypeStr=int16  SampleTime=-1
  Constant2 : Constant  OutDataTypeStr=int16  SampleTime=-1
  Constant3 : Constant  Value=0  OutDataTypeStr=int16  SampleTime=-1
  Constant5 : Constant  Value=-1  OutDataTypeStr=int16  SampleTime=-1
  Detec_edge : Sum  Inputs=+-  AccumDataTypeStr=int8  OutDataTypeStr=int8
  Relational Operator : RelationalOperator  Operator=>  OutDataTypeStr=boolean  RndMeth=Nearest
  Relational Operator1 : RelationalOperator  Operator=<=  OutDataTypeStr=boolean  RndMeth=Nearest
  Reset_flag : Sum  Inputs=+-  AccumDataTypeStr=uint8  OutDataTypeStr=uint8
  Resett_switch1 : Switch  Criteria=u2 ~= 0  OutDataTypeStr=int16
  Resett_switch2 : Switch  Criteria=u2 ~= 0  OutDataTypeStr=int16
  Resett_switch3 : Switch  Criteria=u2 ~= 0  OutDataTypeStr=int16
  only_use_for_neg_speed : Switch  Threshold=1
  reset_old{,1..5} (6 alike) : Delay  DelayLength=1
  reset_old_switch : Switch  Criteria=u2 ~= 0
  reset_old_switch1 : Switch  Criteria=u2 ~= 0
  speed_old_switch1 : Switch  Criteria=u2 ~= 0
  speed_old_switch2 : Switch  Threshold=1
  count : Outport
  wires:
  reset_old5/1 -> only_use_for_neg_speed/2, speed_old_switch2/2
  reset_old4/1 -> speed_old_switch1/1
  only_use_for_neg_speed/1 -> Resett_switch3/2
  Relational Operator1/1 -> only_use_for_neg_speed/3
  reset_old2/1 -> Relational Operator1/1
  Resett_switch2/1 -> Resett_switch3/3
  Resett_switch3/1 -> Resett_switch1/3, reset_old2/1
  Constant1/1 -> Resett_switch1/1, Relational Operator1/2, only_use_for_neg_speed/1, Resett_switch2/1
  Relational Operator/1 -> Resett_switch1/2
  Resett_switch1/1 -> reset_old3/1
  reset_old3/1 -> Relational Operator/1, count/1, Add1/2
  speed_old_switch2/1 -> reset_old4/1
  Constant5/1 -> speed_old_switch2/3
  Dir/1 -> reset_old5/1
  IncsPerTurn/1 -> Relational Operator/2, Resett_switch3/1
  Constant2/1 -> speed_old_switch2/1
  Constant3/1 -> speed_old_switch1/3
  speed_old_switch1/1 -> Add1/1
  Add1/1 -> Resett_switch2/3
  Detec_edge/1 -> reset_old_switch1/2, speed_old_switch1/2  "1 for one cycle if edge recognized"
  reset_old1/1 -> Detec_edge/2, reset_old_switch1/3
  reset_old_switch1/1 -> reset_old1/1
  Enable_ctr/1 -> reset_old_switch1/1, Detec_edge/1
  Reset_flag/1 -> Resett_switch2/2, reset_old_switch/2
  reset_old/1 -> Reset_flag/2, reset_old_switch/3
  reset_old_switch/1 -> reset_old/1
  Reset/1 -> reset_old_switch/1, Reset_flag/1

== system gm_Encoder_Zynq/IncreEncoder_V16/n_aus_theta ==
  count : Inport
  IncsPerTurn : Inport  Port=2
  T : Inport  Port=3
  Add : Sum  Inputs=+-
  Add1 : Sum
  Constant : Constant  Value=0  OutDataTypeStr=fixdt(0,30,24)  SampleTime=-1
  Constant1 : Constant  Value=0  OutDataTypeStr=fixdt(0,30,24)  SampleTime=-1
  Constant2 : Constant  Value=0  OutDataTypeStr=fixdt(0,30,24)  SampleTime=-1
  Gain : Gain  Gain=0.001  ParamDataTypeStr=fixdt(0,16)  OutMin=0  OutMax=0.001*2^16  OutDataTypeStr=fixdt(0,18)
  Product : Product  OutDataTypeStr=Inherit: Same as first input
  ProtectOverflow_T_count : Switch  Threshold=50
  ProtectOverflow_rps : Switch  Threshold=50  OutDataTypeStr=fixdt(0,30,24)
  T_count : Delay  DelayLength=1
  T_count_switch : Switch  Criteria=u2 ~= 0
  count_old : Delay  DelayLength=1
  count_old_switch : Switch  Criteria=u2 ~= 0
  speed_old : Delay  DelayLength=1
  speed_old_switch : Switch  Criteria=u2 ~= 0
  rps : Outport
  wires:
  T_count_switch/1 -> ProtectOverflow_T_count/3, ProtectOverflow_T_count/2, ProtectOverflow_rps/2
  count/1 -> count_old_switch/1, Add/1
  Add1/1 -> T_count_switch/3, Product/1
  Product/1 -> speed_old_switch/1
  T_count/1 -> Add1/2
  ProtectOverflow_T_count/1 -> T_count/1
  T/1 -> Add1/1
  Gain/1 -> Product/2
  IncsPerTurn/1 -> Gain/1
  speed_old/1 -> speed_old_switch/3
  speed_old_switch/1 -> speed_old/1, ProtectOverflow_rps/3
  Constant2/1 -> ProtectOverflow_rps/1
  ProtectOverflow_rps/1 -> rps/1
  Constant1/1 -> ProtectOverflow_T_count/1
  Add/1 -> T_count_switch/2, count_old_switch/2, speed_old_switch/2
  Constant/1 -> T_count_switch/1
  count_old/1 -> Add/2, count_old_switch/3
  count_old_switch/1 -> count_old/1

== system gm_Encoder_Zynq/IncreEncoder_V18/Check_Direction ==
  A : Inport
  B : Inport  Port=2
  Add : Sum  Inputs=+-  AccumDataTypeStr=fixdt(1,4,0)  OutDataTypeStr=fixdt(1,4,0)
  Add1 : Sum  Inputs=+-  AccumDataTypeStr=fixdt(1,4,0)  OutDataTypeStr=fixdt(1,4,0)
  Add2 : Sum  AccumDataTypeStr=fixdt(1,4,0)  OutDataTypeStr=fixdt(1,4,0)
  Change : Sum  AccumDataTypeStr=fixdt(1,4,0)  OutDataTypeStr=fixdt(1,4,0)
  Change1 : Delay  DelayLength=1
  Save_Direction : Switch  Criteria=u2 ~= 0  Threshold=0.1  OutDataTypeStr=Inherit: Inherit via back propagation
  Scope6 : Scope  NumInputPorts=4
  T_count_switch : Switch  Threshold=1  OutDataTypeStr=Inherit: Inherit via back propagation
  TrnLeft : Sum  Inputs=+-  AccumDataTypeStr=fixdt(1,4,0)  OutDataTypeStr=fixdt(1,4,0)
  TrnRight : Sum  Inputs=+-  AccumDataTypeStr=fixdt(1,4,0)  OutDataTypeStr=fixdt(1,4,0)
  TurnLeft : Constant  Value=-1  OutDataTypeStr=fixdt(1,4,0)  SampleTime=-1
  TurnRight : Constant  OutDataTypeStr=fixdt(1,4,0)  SampleTime=-1
  count_old : Delay  DelayLength=1
  count_old1 : Delay  DelayLength=1
  count_old2 : Delay  DelayLength=1
  count_old_switch : Switch  Criteria=u2 ~= 0  OutDataTypeStr=Inherit: Inherit via back propagation
  count_old_switch1 : Switch  Criteria=u2 ~= 0  OutDataTypeStr=Inherit: Inherit via back propagation
  new_value : Delay  DelayLength=1
  nothing : Constant  Value=0  OutDataTypeStr=fixdt(1,4,0)  SampleTime=-1
  nothing1 : Constant  Value=0  OutDataTypeStr=fixdt(1,4,0)  SampleTime=-1
  speed_old_switch : Switch  Threshold=1  OutDataTypeStr=Inherit: Inherit via back propagation
  Dir : Outport
  wires:
  count_old2/1 -> Dir/1, Save_Direction/3
  Change1/1 -> Save_Direction/2, Scope6/3
  Change/1 -> Change1/1
  Add2/1 -> new_value/1, Scope6/4
  speed_old_switch/1 -> Add2/2, Change/2
  nothing1/1 -> T_count_switch/3
  nothing/1 -> speed_old_switch/3
  TurnLeft/1 -> speed_old_switch/1
  TrnLeft/1 -> Scope6/2, speed_old_switch/2
  new_value/1 -> Save_Direction/1
  TrnRight/1 -> T_count_switch/2, Scope6/1
  Add1/1 -> count_old_switch1/2, TrnLeft/1
  count_old1/1 -> Add1/2, count_old_switch1/3
  count_old_switch1/1 -> count_old1/1
  B/1 -> count_old_switch1/1, Add1/1, TrnRight/2
  Save_Direction/1 -> count_old2/1
  T_count_switch/1 -> Add2/1, Change/1
  Add/1 -> count_old_switch/2, TrnRight/1
  TurnRight/1 -> T_count_switch/1
  count_old/1 -> Add/2, count_old_switch/3
  count_old_switch/1 -> count_old/1
  A/1 -> count_old_switch/1, Add/1, TrnLeft/2

== system gm_Encoder_Zynq/IncreEncoder_V18/Counter_speed ==
  note: Count
  note: Reset
  note: Check if count is to big
  note: Check if count is to small
  note: 1 for one cycle if edge recognized
  Enable_ctr : Inport
  Reset : Inport  Port=2
  IncsPerTurn : Inport  Port=3
  Add1 : Sum  AccumDataTypeStr=int16  OutDataTypeStr=uint16
  Constant1 : Constant  Value=0  OutDataTypeStr=uint16  SampleTime=-1
  Constant2 : Constant  OutDataTypeStr=int8  SampleTime=-1
  Constant3 : Constant  Value=0  OutDataTypeStr=int8  SampleTime=-1
  Constant4 : Constant  Value=10  OutDataTypeStr=uint16  SampleTime=-1
  Detec_edge : Sum  Inputs=+-  AccumDataTypeStr=int8  OutDataTypeStr=int8
  Relational Operator : RelationalOperator  OutDataTypeStr=boolean  RndMeth=Nearest
  Reset_flag : Sum  Inputs=+-  AccumDataTypeStr=uint8  OutDataTypeStr=uint8
  Reset_when_overflow : Sum
  Resett_switch1 : Switch  Criteria=u2 ~= 0
  Resett_switch2 : Switch  Criteria=u2 ~= 0
  reset_old{,1..3} (4 alike) : Delay  DelayLength=1
  reset_old_switch : Switch  Criteria=u2 ~= 0
  reset_old_switch1 : Switch  Criteria=u2 ~= 0
  speed_old_switch1 : Switch  Threshold=1
  count : Outport
  wires:
  reset_old3/1 -> Relational Operator/2
  Resett_switch2/1 -> Resett_switch1/3
  IncsPerTurn/1 -> Reset_when_overflow/2
  Constant1/1 -> Resett_switch1/1, Resett_switch2/1
  Relational Operator/1 -> Resett_switch1/2
  Resett_switch1/1 -> reset_old2/1
  Reset_when_overflow/1 -> reset_old3/1
  Constant4/1 -> Reset_when_overflow/1
  Constant2/1 -> speed_old_switch1/1
  Constant3/1 -> speed_old_switch1/3
  speed_old_switch1/1 -> Add1/1
  reset_old2/1 -> count/1, Add1/2, Relational Operator/1
  Add1/1 -> Resett_switch2/3
  Detec_edge/1 -> reset_old_switch1/2, speed_old_switch1/2  "1 for one cycle if edge recognized"
  reset_old1/1 -> Detec_edge/2, reset_old_switch1/3
  reset_old_switch1/1 -> reset_old1/1
  Enable_ctr/1 -> reset_old_switch1/1, Detec_edge/1
  Reset_flag/1 -> Resett_switch2/2, reset_old_switch/2
  reset_old/1 -> Reset_flag/2, reset_old_switch/3
  reset_old_switch/1 -> reset_old/1
  Reset/1 -> reset_old_switch/1, Reset_flag/1

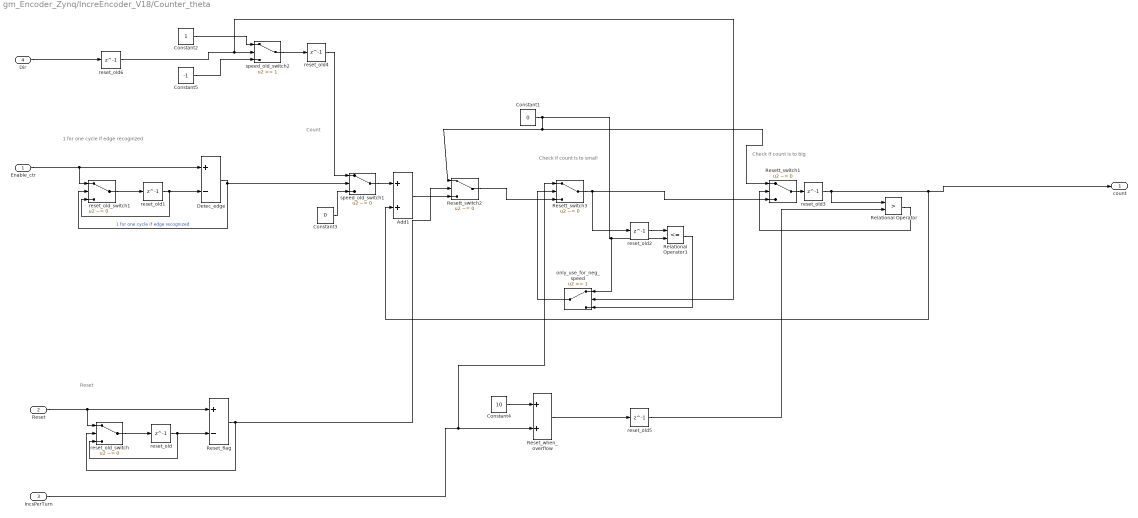
== system gm_Encoder_Zynq/IncreEncoder_V18/Counter_theta ==
  note: Check if count is to small
  note: Check if count is to big
  note: Count
  note: Reset
  note: 1 for one cycle if edge recognized
  Enable_ctr : Inport
  Reset : Inport  Port=2
  IncsPerTurn : Inport  Port=3
  Dir : Inport  Port=4
  Add1 : Sum  AccumDataTypeStr=int16  OutDataTypeStr=int16
  Constant1 : Constant  Value=0  OutDataTypeStr=int16  SampleTime=-1
  Constant2 : Constant  OutDataTypeStr=int16  SampleTime=-1
  Constant3 : Constant  Value=0  OutDataTypeStr=int16  SampleTime=-1
  Constant4 : Constant  Value=10  OutDataTypeStr=int16  SampleTime=-1
  Constant5 : Constant  Value=-1  OutDataTypeStr=int16  SampleTime=-1
  Detec_edge : Sum  Inputs=+-  AccumDataTypeStr=int8  OutDataTypeStr=int8
  Relational Operator : RelationalOperator  Operator=>  OutDataTypeStr=boolean  RndMeth=Nearest
  Relational Operator1 : RelationalOperator  Operator=<=  OutDataTypeStr=boolean  RndMeth=Nearest
  Reset_flag : Sum  Inputs=+-  AccumDataTypeStr=uint8  OutDataTypeStr=uint8
  Reset_when_overflow : Sum  OutDataTypeStr=int16
  Resett_switch1 : Switch  Criteria=u2 ~= 0  OutDataTypeStr=int16
  Resett_switch2 : Switch  Criteria=u2 ~= 0  OutDataTypeStr=int16
  Resett_switch3 : Switch  Criteria=u2 ~= 0  OutDataTypeStr=int16
  only_use_for_neg_speed : Switch  Threshold=1
  reset_old{,1..6} (7 alike) : Delay  DelayLength=1
  reset_old_switch : Switch  Criteria=u2 ~= 0
  reset_old_switch1 : Switch  Criteria=u2 ~= 0
  speed_old_switch1 : Switch  Criteria=u2 ~= 0
  speed_old_switch2 : Switch  Threshold=1
  count : Outport
  wires:
  reset_old6/1 -> speed_old_switch2/2, only_use_for_neg_speed/2
  reset_old5/1 -> Relational Operator/2
  reset_old4/1 -> speed_old_switch1/1
  only_use_for_neg_speed/1 -> Resett_switch3/2
  Relational Operator1/1 -> only_use_for_neg_speed/3
  reset_old2/1 -> Relational Operator1/1
  Resett_switch2/1 -> Resett_switch3/3
  Resett_switch3/1 -> Resett_switch1/3, reset_old2/1
  Constant1/1 -> Relational Operator1/2, only_use_for_neg_speed/1, Resett_switch1/1, Resett_switch2/1
  Relational Operator/1 -> Resett_switch1/2
  Resett_switch1/1 -> reset_old3/1
  reset_old3/1 -> Relational Operator/1, count/1, Add1/2
  speed_old_switch2/1 -> reset_old4/1
  Constant5/1 -> speed_old_switch2/3
  Dir/1 -> reset_old6/1
  IncsPerTurn/1 -> Reset_when_overflow/2, Resett_switch3/1
  Reset_when_overflow/1 -> reset_old5/1
  Constant4/1 -> Reset_when_overflow/1
  Constant2/1 -> speed_old_switch2/1
  Constant3/1 -> speed_old_switch1/3
  speed_old_switch1/1 -> Add1/1
  Add1/1 -> Resett_switch2/3
  Detec_edge/1 -> reset_old_switch1/2, speed_old_switch1/2  "1 for one cycle if edge recognized"
  reset_old1/1 -> Detec_edge/2, reset_old_switch1/3
  reset_old_switch1/1 -> reset_old1/1
  Enable_ctr/1 -> reset_old_switch1/1, Detec_edge/1
  Reset_flag/1 -> Resett_switch2/2, reset_old_switch/2
  reset_old/1 -> Reset_flag/2, reset_old_switch/3
  reset_old_switch/1 -> reset_old/1
  Reset/1 -> reset_old_switch/1, Reset_flag/1
